simulink model "untitled1_no_noise"  (R2018b)
settings: Solver=VariableStepAuto  StartTime=0.0  StopTime=0.5  RelTol=1e-3
libraries: commblksprivate x2, commutil2 x2, dsparch4 x1
settings Model: Creator=43724  LastModifiedBy=43724
settings DataIOCC: LimitDataPoints=on  Refine=200

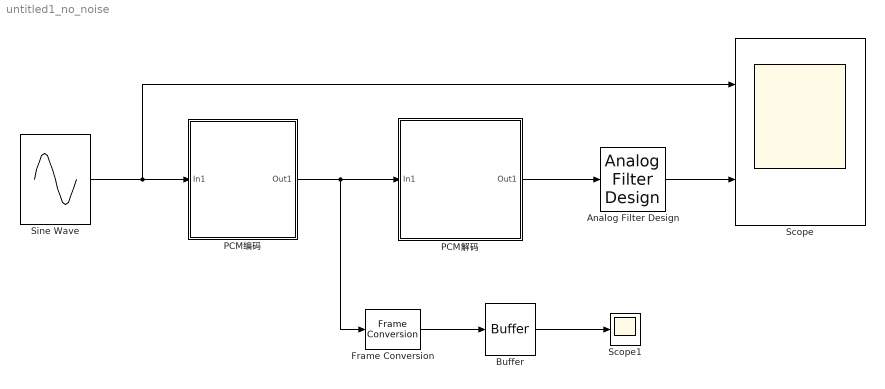
== system untitled1_no_noise ==
  Analog Filter Design : dsparch4/Analog Filter Design  method=Butterworth  filttype=Lowpass  N=8  Wlo=250*pi  Whi=80  Rp=2  Rs=40
  Buffer : Buffer  N=1  OutputFrames=off
  Frame Conversion : FrameConversion
  PCM编码 : Subsystem
  PCM解码 : Subsystem
  Scope : Scope  NumInputPorts=2
  Scope1 : Scope
  Sine Wave : Sin  Frequency=200*pi  SampleTime=0
  wires:
  Sine Wave/1 -> Scope/1, PCM编码/1(In1)
  PCM编码/1(Out1) -> PCM解码/1(In1), Frame Conversion/1
  PCM解码/1(Out1) -> Analog Filter Design/1
  Analog Filter Design/1 -> Scope/2
  Frame Conversion/1 -> Buffer/1
  Buffer/1 -> Scope1/1

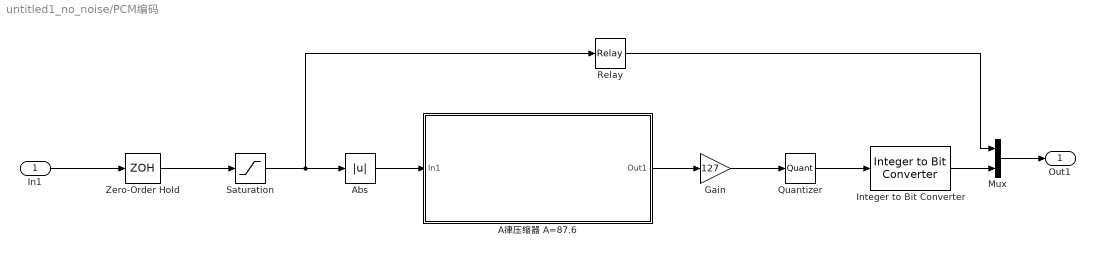
== system untitled1_no_noise/PCM编码 ==
  In1 : Inport
  Abs : Abs
  A律压缩器 A=87.6 : Subsystem
  Gain : Gain  Gain=127
  Integer to Bit Converter : commutil2/Integer to Bit Converter  nbits=7  signedInputValues=Unsigned  bitOrder=MSB first  outDtype=Inherit via internal rule
  Mux : Mux  Inputs=2
  Quantizer : Quantizer  QuantizationInterval=1
  Relay : Relay
  Saturation : Saturate  UpperLimit=1  LowerLimit=-1
  Zero-Order Hold : ZeroOrderHold  SampleTime=0.001
  Out1 : Outport
  wires:
  Quantizer/1 -> Integer to Bit Converter/1
  Mux/1 -> Out1/1
  Integer to Bit Converter/1 -> Mux/2
  Saturation/1 -> Relay/1, Abs/1
  Gain/1 -> Quantizer/1
  Relay/1 -> Mux/1
  In1/1 -> Zero-Order Hold/1
  Zero-Order Hold/1 -> Saturation/1
  Abs/1 -> A律压缩器 A=87.6/1(In1)
  A律压缩器 A=87.6/1(Out1) -> Gain/1

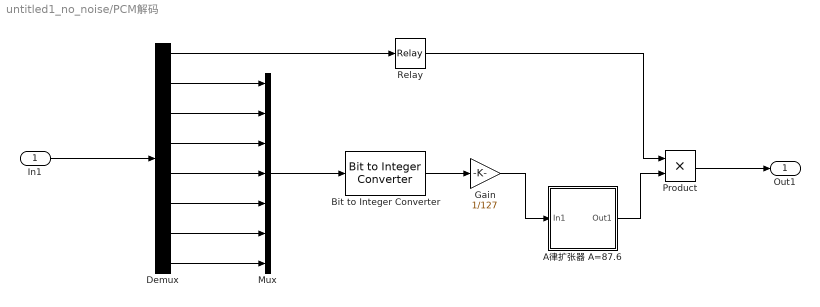
== system untitled1_no_noise/PCM解码 ==
  In1 : Inport
  "A律扩张器 A=87.6 " : Subsystem
  Bit to Integer Converter : commutil2/Bit to Integer Converter  nbits=7  bitOrder=MSB first  signedOutputValues=Unsigned  outDtype=Inherit via internal rule  outDtypeSigned=Inherit via internal rule
  Demux : Demux  Outputs=8
  Gain : Gain  Gain=1/127
  Mux : Mux  Inputs=7
  Product : Product
  Relay : Relay  OffOutputValue=-1
  Out1 : Outport
  wires:
  Demux/1 -> Relay/1
  Demux/8 -> Mux/7
  In1/1 -> Demux/1
  Demux/2 -> Mux/1
  Demux/7 -> Mux/6
  Mux/1 -> Bit to Integer Converter/1
  Demux/5 -> Mux/4
  Demux/4 -> Mux/3
  Demux/3 -> Mux/2
  Product/1 -> Out1/1
  Bit to Integer Converter/1 -> Gain/1
  Relay/1 -> Product/1
  Demux/6 -> Mux/5
  Gain/1 -> "A律扩张器 A=87.6 "/1(In1)
  "A律扩张器 A=87.6 "/1(Out1) -> Product/2

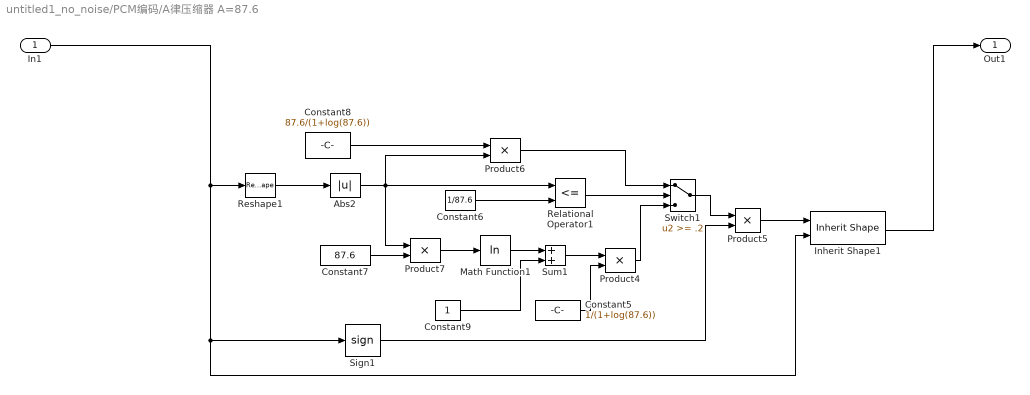
== system untitled1_no_noise/PCM编码/A律压缩器 A=87.6 ==
  In1 : Inport
  Abs2 : Abs  SaturateOnIntegerOverflow=on
  Constant5 : Constant  Value=1/(1+log(87.6))
  Constant6 : Constant  Value=1/87.6
  Constant7 : Constant  Value=87.6
  Constant8 : Constant  Value=87.6/(1+log(87.6))
  Constant9 : Constant
  Inherit Shape1 : commblksprivate/Inherit Shape
      settings: SourceProductName=Communications System Toolbox  SourceProductBaseCode=CM
  Math Function1 : Math  Operator=log  SaturateOnIntegerOverflow=on
  Product{4..7} (4 alike) : Product  SaturateOnIntegerOverflow=on  InputSameDT=on  OutDataTypeStr=Inherit: Same as first input
  Relational Operator1 : RelationalOperator  Operator=<=  OutDataTypeStr=float('double')  RndMeth=Nearest  InputSameDT=on
  Reshape1 : Reshape
  Sign1 : Signum
  Sum1 : Sum  SaturateOnIntegerOverflow=on  InputSameDT=on  OutDataTypeStr=Inherit: Same as first input
  Switch1 : Switch  Threshold=.2  SaturateOnIntegerOverflow=on  InputSameDT=on
  Out1 : Outport
  wires:
  Sum1/1 -> Product4/1
  Abs2/1 -> Relational Operator1/1, Product6/2, Product7/1
  Constant9/1 -> Sum1/2
  Switch1/1 -> Product5/1
  Product4/1 -> Switch1/3
  Sign1/1 -> Product5/2
  Product6/1 -> Switch1/1
  In1/1 -> Inherit Shape1/2, Sign1/1, Reshape1/1
  Constant8/1 -> Product6/1
  Constant5/1 -> Product4/2
  Reshape1/1 -> Abs2/1
  Constant6/1 -> Relational Operator1/2
  Relational Operator1/1 -> Switch1/2
  Math Function1/1 -> Sum1/1
  Product7/1 -> Math Function1/1
  Constant7/1 -> Product7/2
  Product5/1 -> Inherit Shape1/1
  Inherit Shape1/1 -> Out1/1

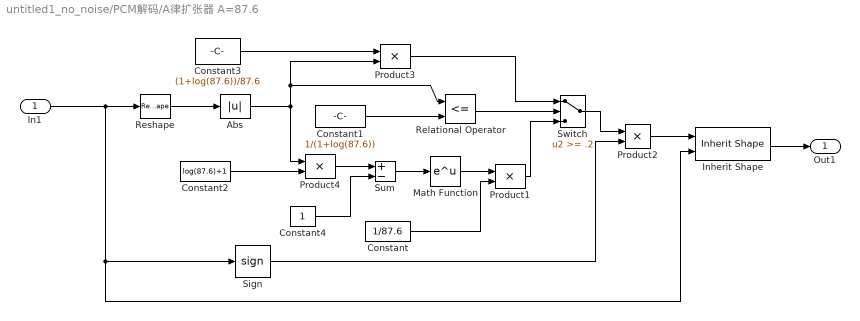
== system untitled1_no_noise/PCM解码/A律扩张器 A=87.6  ==
  In1 : Inport
  Abs : Abs  SaturateOnIntegerOverflow=on
  Constant : Constant  Value=1/87.6
  Constant1 : Constant  Value=1/(1+log(87.6))
  Constant2 : Constant  Value=log(87.6)+1
  Constant3 : Constant  Value=(1+log(87.6))/87.6
  Constant4 : Constant
  Inherit Shape : commblksprivate/Inherit Shape
      settings: SourceProductName=Communications System Toolbox  SourceProductBaseCode=CM
  Math Function : Math  SaturateOnIntegerOverflow=on
  Product{1..4} (4 alike) : Product  SaturateOnIntegerOverflow=on  InputSameDT=on  OutDataTypeStr=Inherit: Same as first input
  Relational Operator : RelationalOperator  Operator=<=  OutDataTypeStr=float('double')  RndMeth=Nearest  InputSameDT=on
  Reshape : Reshape
  Sign : Signum
  Sum : Sum  Inputs=+-  SaturateOnIntegerOverflow=on  InputSameDT=on  OutDataTypeStr=Inherit: Same as first input
  Switch : Switch  Threshold=.2  SaturateOnIntegerOverflow=on  InputSameDT=on
  Out1 : Outport
  wires:
  Constant3/1 -> Product3/1
  In1/1 -> Sign/1, Inherit Shape/2, Reshape/1
  Sum/1 -> Math Function/1
  Product2/1 -> Inherit Shape/1
  Product1/1 -> Switch/3
  Reshape/1 -> Abs/1
  Constant2/1 -> Product4/2
  Switch/1 -> Product2/1
  Constant/1 -> Product1/2
  Math Function/1 -> Product1/1
  Abs/1 -> Relational Operator/1, Product3/2, Product4/1
  Constant4/1 -> Sum/2
  Constant1/1 -> Relational Operator/2
  Product4/1 -> Sum/1
  Product3/1 -> Switch/1
  Sign/1 -> Product2/2
  Relational Operator/1 -> Switch/2
  Inherit Shape/1 -> Out1/1
